simulink model "GRAY"  (R2019b)
settings: Solver=VariableStepAuto  StartTime=0.0  StopTime=10.0  RelTol=1e-3
libraries: simulink x4
settings Model: Creator=simone  LastModifiedBy=simone

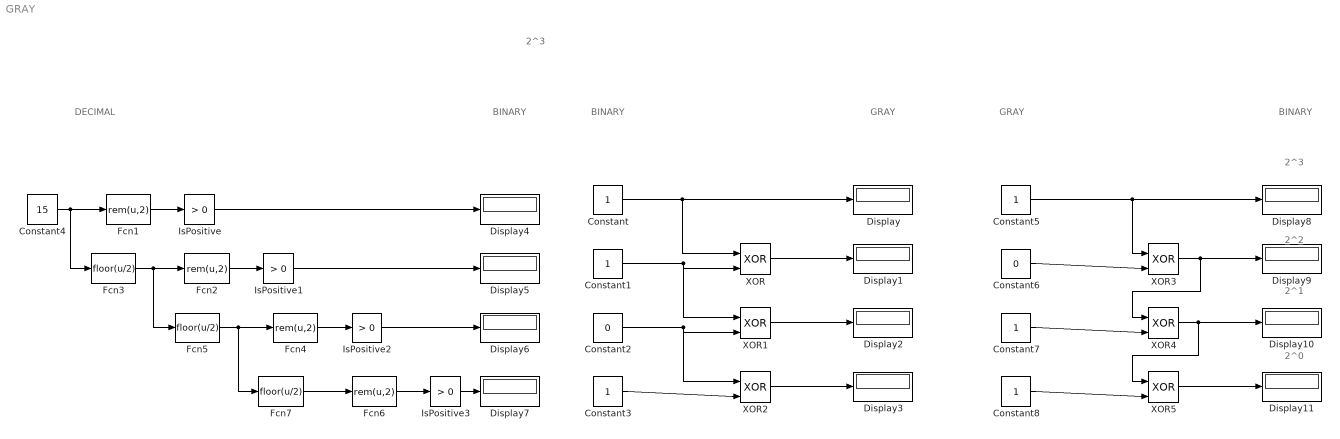
== system GRAY ==
  note: 2^3
  note: DECIMAL
  note: GRAY
  note: BINARY
  note: BINARY
  note: BINARY
  note: GRAY
  note: 2^3
  note: 2^2
  note: 2^1
  note: 2^0
  Constant{,1,3,5,7..8} (6 alike) : Constant
  Constant2 : Constant  Value=0
  Constant4 : Constant  Value=15
  Constant6 : Constant  Value=0
  Display{,1..11} (12 alike) : Display
  Fcn{1..2,4,6} (4 alike) : Fcn  Expr=rem(u,2)
  Fcn3 : Fcn  Expr=floor(u/2)
  Fcn5 : Fcn  Expr=floor(u/2)
  Fcn7 : Fcn  Expr=floor(u/2)
  IsPositive{,1..3} (4 alike) : simulink/Logic and Bit Operations/Compare To Zero  relop=>  OutDataTypeStr=boolean
  XOR{,1..5} (6 alike) : Logic  Operator=XOR  IconShape=distinctive  AllPortsSameDT=off  OutDataTypeStr=boolean
  wires:
  Constant/1 -> XOR/1, Display/1
  XOR/1 -> Display1/1
  Constant2/1 -> XOR2/1, XOR1/2
  XOR1/1 -> Display2/1
  Constant3/1 -> XOR2/2
  XOR2/1 -> Display3/1
  IsPositive/1 -> Display4/1
  Constant4/1 -> Fcn3/1, Fcn1/1
  Fcn3/1 -> Fcn2/1, Fcn5/1
  Fcn7/1 -> Fcn6/1
  Fcn5/1 -> Fcn4/1, Fcn7/1
  Fcn1/1 -> IsPositive/1
  Fcn2/1 -> IsPositive1/1
  IsPositive1/1 -> Display5/1
  Fcn4/1 -> IsPositive2/1
  IsPositive2/1 -> Display6/1
  Fcn6/1 -> IsPositive3/1
  IsPositive3/1 -> Display7/1
  Constant6/1 -> XOR3/2
  Constant5/1 -> XOR3/1, Display8/1
  XOR3/1 -> XOR4/1, Display9/1
  Constant8/1 -> XOR5/2
  Constant7/1 -> XOR4/2
  XOR4/1 -> XOR5/1, Display10/1
  XOR5/1 -> Display11/1
  Constant1/1 -> XOR1/1, XOR/2
